simulink model "CounterStateflow"  (R2020b)
settings: Solver=VariableStepAuto  StartTime=0.0  StopTime=10.0  RelTol=1e-3
settings Model: EnablePacing=on  PacingRate=0.220000  Creator=lenovo  LastModifiedBy=lenovo

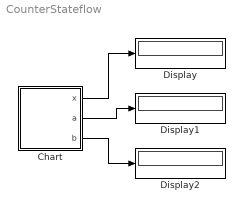
== system CounterStateflow ==
  Chart : Stateflow chart  TreatAsAtomicUnit=on
  Display : Display
  Display1 : Display
  Display2 : Display
  wires:
  Chart/1(x) -> Display/1
  Chart/2(a) -> Display1/1
  Chart/3(b) -> Display2/1

== stateflow chart CounterStateflow/Chart ==
  state Counter_UnitDIgit
    entry:
    x=0;
    during:
    x=x+1;
  state initiate_values
    entry:
    a=0
    b=0;
  state Tens_digit
    entry:
    during:
    a=a+1;
  state Hundred_digit
    entry:
    during:
    b=b+1;
  state END
  (default) -> initiate_values
  initiate_values -> Counter_UnitDIgit
  (junction 84) -> Counter_UnitDIgit [order 2] : {a~=5}
  Counter_UnitDIgit -> Tens_digit : [x==5]
  (junction 100) -> Tens_digit [order 2] : {b~=5}
  Tens_digit -> (junction 84) : [a]
  (junction 84) -> Hundred_digit [order 1] : [a==5]
  Hundred_digit -> (junction 100) : [b]
  (junction 100) -> END [order 1] : [b==5]
  data: x output size=1; a output; z1 constant double; b output
